simulink model "HWR"  (R2022b)
settings: Solver=ode23t  StartTime=0.0  StopTime=0.08  RelTol=1e-3
libraries: dspsigops x5, simulink x2, spsSeriesRLCBranchLib x2, spsVoltageMeasurementLib x2, spsACVoltageSourceLib x1, spsCurrentMeasurementLib x1, spspowerguiLib x1
settings Model: Creator=HP  LastModifiedBy=HP

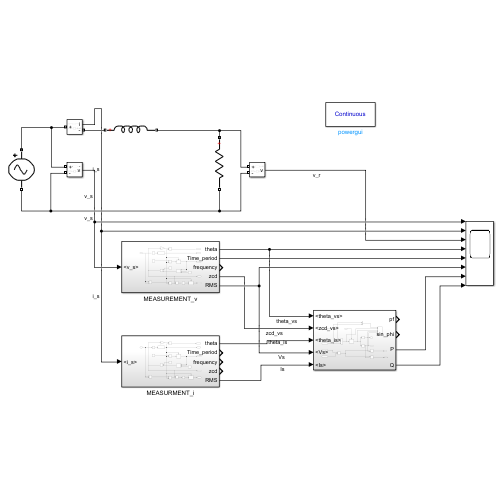
[thumbnail: Simulink's stored preview of the top-level diagram]
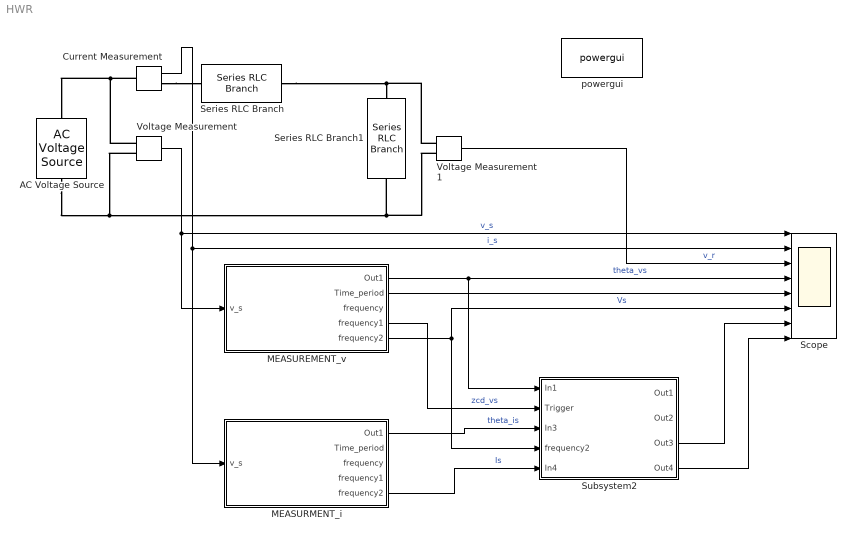
== system HWR ==
  AC Voltage Source : spsACVoltageSourceLib/AC Voltage Source  Amplitude=230*sqrt(2)  Phase=0  Frequency=1000  SampleTime=0  Measurements=None  BusType=swing  Pref=10e3  Qref=0  Qmin=-inf  Qmax=+inf
  Current Measurement : spsCurrentMeasurementLib/Current Measurement  PhasorSimulation=off  OutputType=Complex  PSBequivalent=0
  MEASUREMENT_v : Subsystem
  MEASURMENT_i : Subsystem
  Scope : Scope  NumInputPorts=8
  Series RLC Branch : spsSeriesRLCBranchLib/Series RLC Branch  LConnTagsString=__new0  RConnTagsString=__new0  BranchType=L  Resistance=1  Inductance=12.7e-3  SetiL0=off  InitialCurrent=0  Capacitance=1e-6  Setx0=off  InitialVoltage=0  Measurements=None
  Series RLC Branch1 : spsSeriesRLCBranchLib/Series RLC Branch  LConnTagsString=__new0  RConnTagsString=__new0  BranchType=R  Resistance=10  Inductance=12.7e-3  SetiL0=off  InitialCurrent=0  Capacitance=1e-6  Setx0=off  InitialVoltage=0  Measurements=None
  Subsystem2 : Subsystem
  Voltage Measurement : spsVoltageMeasurementLib/Voltage Measurement  PhasorSimulation=off  OutputType=Complex  PSBequivalent=0
  Voltage Measurement1 : spsVoltageMeasurementLib/Voltage Measurement  PhasorSimulation=off  OutputType=Complex  PSBequivalent=0
  powergui : spspowerguiLib/powergui  Priority=1  SimulationMode=Continuous  SampleTime=50e-6  frequency=60  Iterations=50  frequencyindice=1000  Pbase=100e6  ErrMax=1e-4  UnitsV=kV  UnitsW=MW  buscounter=0  FunctionMessages=off  echomessages=off  EnableUseOfTLC=off  CurrentSourceSwitches=off  DisableSnubberDevices=off  DisableRonSwitches=off  DisableVfSwitches=off  DisplayEquations=off  AutomaticDiscreteSolvers=off  SolverType=Tustin/Backward Euler (TBE)  Interpol=off  ExternalGateDelay=off  methode=off  Ts=100  x0status=blocks  SPID=on  SwTol=0  HookPort=off  NonlinearTolerance=1e-4  nMaxIteration=100  ContinueOnMaxIteration=off  RestoreLinks=warning  ResistiveCurrentMeasurement=off  Frange=[0:2:500]  Ylog=off  Xlog=on  ShowGrid=off  save=off  variable=ZData  structure=0  ZoomFFT=off  StartTime=0.0  cycles=1  DisplayStyle=1  fundamental=60  FreqAxis=off  MaxFrequency=1000  frequencyindicesteady=1  RmsSteady=1  display=off
  wires:
  Voltage Measurement/1 -> MEASUREMENT_v/1(v_s), Scope/1  "v_s"
  Current Measurement/1 -> MEASURMENT_i/1(v_s), Scope/2  "i_s"
  Voltage Measurement1/1 -> Scope/3  "v_r"
  MEASUREMENT_v/1(Out1) -> Subsystem2/1(In1), Scope/4  "theta_vs"
  MEASUREMENT_v/2(Time_period) -> Scope/5
  MEASUREMENT_v/5(frequency2) -> Subsystem2/4(frequency2), Scope/6  "Vs"
  MEASUREMENT_v/4(frequency1) -> Subsystem2/2(Trigger)  "zcd_vs"
  MEASURMENT_i/1(Out1) -> Subsystem2/3(In3)  "theta_is"
  MEASURMENT_i/5(frequency2) -> Subsystem2/5(In4)  "Is"
  Subsystem2/3(Out3) -> Scope/7
  Subsystem2/4(Out4) -> Scope/8
  connections:
  AC Voltage Source/LConn1 -- Voltage Measurement1/LConn2 -- Series RLC Branch1/RConn1 -- Voltage Measurement/LConn2
  Series RLC Branch/RConn1 -- Voltage Measurement1/LConn1 -- Series RLC Branch1/LConn1
  Current Measurement/RConn1 -- Series RLC Branch/LConn1
  Current Measurement/LConn1 -- Voltage Measurement/LConn1 -- AC Voltage Source/RConn1

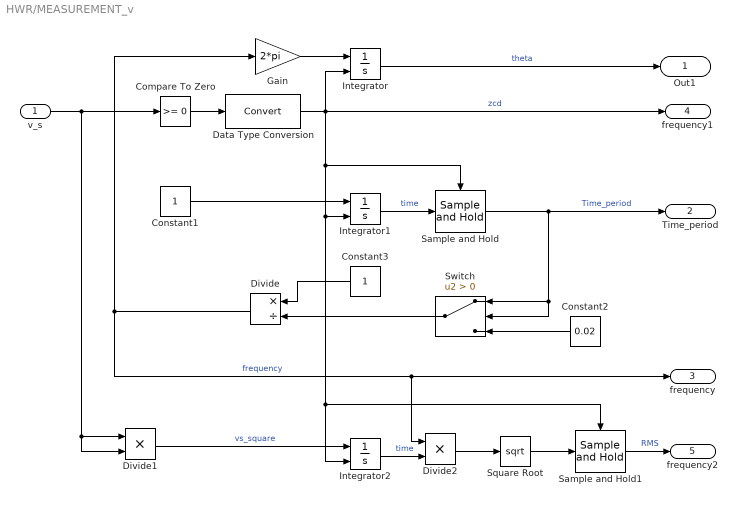
== system HWR/MEASUREMENT_v ==
  v_s : Inport
  Compare To Zero : simulink/Logic and Bit Operations/Compare To Zero  relop=>=  OutDataTypeStr=boolean
  Constant1 : Constant
  Constant2 : Constant  Value=0.02
  Constant3 : Constant
  Data Type Conversion : DataTypeConversion  SaturateOnIntegerOverflow=off  RndMeth=Floor
  Divide : Product  Inputs=*/
  Divide1 : Product  Inputs=**
  Divide2 : Product  Inputs=**
  Gain : Gain  Gain=2*pi
  Integrator : Integrator  ExternalReset=rising
  Integrator1 : Integrator  ExternalReset=rising
  Integrator2 : Integrator  ExternalReset=rising
  Sample and Hold : dspsigops/Sample and Hold  trig=Rising edge  initCond=0  latchinput=on
  Sample and Hold1 : dspsigops/Sample and Hold  trig=Rising edge  initCond=0  latchinput=on
  Square Root : Sqrt
  Switch : Switch  Criteria=u2 > Threshold  SaturateOnIntegerOverflow=off  InputSameDT=off
  Out1 : Outport
  Time_period : Outport  Port=2
  frequency : Outport  Port=3
  frequency1 : Outport  Port=4
  frequency2 : Outport  Port=5
  wires:
  Compare To Zero/1 -> Data Type Conversion/1
  Constant3/1 -> Divide/1
  Integrator/1 -> Out1/1  "theta"
  Divide/1 -> Gain/1, Divide2/1, frequency/1  "frequency"
  Data Type Conversion/1 -> Integrator1/2, Sample and Hold1/Trigger, Integrator2/2, Sample and Hold/Trigger, frequency1/1, Integrator/2  "zcd"
  Gain/1 -> Integrator/1
  Sample and Hold/1 -> Time_period/1, Switch/2, Switch/1  "Time_period"
  Constant2/1 -> Switch/3
  Constant1/1 -> Integrator1/1
  Integrator1/1 -> Sample and Hold/1  "time"
  Switch/1 -> Divide/2
  v_s/1 -> Divide1/2, Divide1/1, Compare To Zero/1
  Divide1/1 -> Integrator2/1  "vs_square"
  Integrator2/1 -> Divide2/2  "time"
  Divide2/1 -> Square Root/1
  Square Root/1 -> Sample and Hold1/1
  Sample and Hold1/1 -> frequency2/1  "RMS"

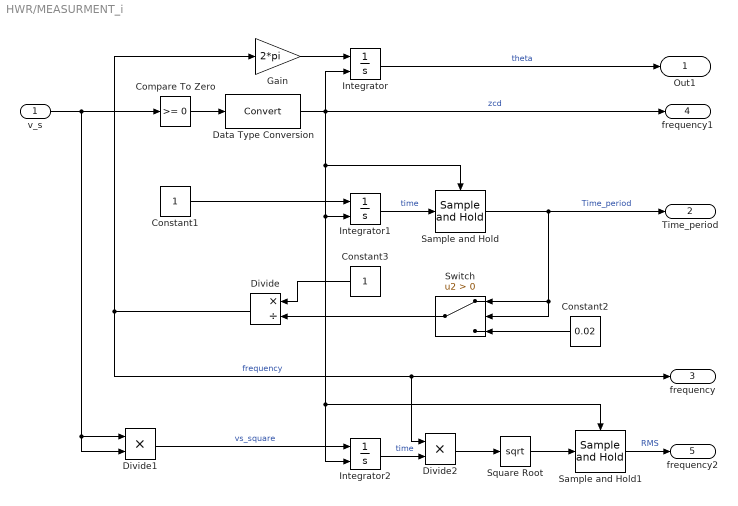
== system HWR/MEASURMENT_i ==
  v_s : Inport
  Compare To Zero : simulink/Logic and Bit Operations/Compare To Zero  relop=>=  OutDataTypeStr=boolean
  Constant1 : Constant
  Constant2 : Constant  Value=0.02
  Constant3 : Constant
  Data Type Conversion : DataTypeConversion  SaturateOnIntegerOverflow=off  RndMeth=Floor
  Divide : Product  Inputs=*/
  Divide1 : Product  Inputs=**
  Divide2 : Product  Inputs=**
  Gain : Gain  Gain=2*pi
  Integrator : Integrator  ExternalReset=rising
  Integrator1 : Integrator  ExternalReset=rising
  Integrator2 : Integrator  ExternalReset=rising
  Sample and Hold : dspsigops/Sample and Hold  trig=Rising edge  initCond=0  latchinput=on
  Sample and Hold1 : dspsigops/Sample and Hold  trig=Rising edge  initCond=0  latchinput=on
  Square Root : Sqrt
  Switch : Switch  Criteria=u2 > Threshold  SaturateOnIntegerOverflow=off  InputSameDT=off
  Out1 : Outport
  Time_period : Outport  Port=2
  frequency : Outport  Port=3
  frequency1 : Outport  Port=4
  frequency2 : Outport  Port=5
  wires:
  Sample and Hold1/1 -> frequency2/1  "RMS"
  Square Root/1 -> Sample and Hold1/1
  Divide2/1 -> Square Root/1
  Integrator2/1 -> Divide2/2  "time"
  Divide1/1 -> Integrator2/1  "vs_square"
  v_s/1 -> Compare To Zero/1, Divide1/1, Divide1/2
  Switch/1 -> Divide/2
  Integrator1/1 -> Sample and Hold/1  "time"
  Constant1/1 -> Integrator1/1
  Constant2/1 -> Switch/3
  Sample and Hold/1 -> Switch/1, Switch/2, Time_period/1  "Time_period"
  Gain/1 -> Integrator/1
  Data Type Conversion/1 -> Integrator/2, frequency1/1, Sample and Hold/Trigger, Integrator2/2, Sample and Hold1/Trigger, Integrator1/2  "zcd"
  Divide/1 -> frequency/1, Divide2/1, Gain/1  "frequency"
  Integrator/1 -> Out1/1  "theta"
  Constant3/1 -> Divide/1
  Compare To Zero/1 -> Data Type Conversion/1

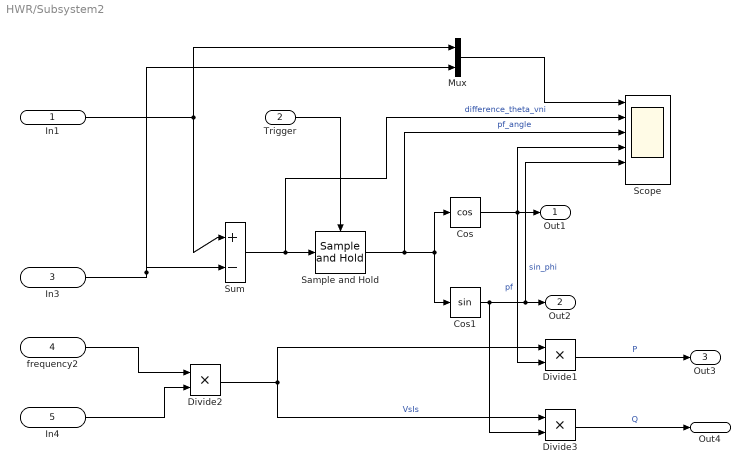
== system HWR/Subsystem2 ==
  In1 : Inport
  Trigger : Inport  Port=2
  In3 : Inport  Port=3
  frequency2 : Inport  Port=4
  In4 : Inport  Port=5
  Cos : Trigonometry  Operator=cos
  Cos1 : Trigonometry
  Divide1 : Product  Inputs=**
  Divide2 : Product  Inputs=**
  Divide3 : Product  Inputs=**
  Mux : Mux  Inputs=2
  Sample and Hold : dspsigops/Sample and Hold  trig=Rising edge  initCond=0  latchinput=on
  Scope : Scope  NumInputPorts=6
  Sum : Sum  Inputs=|+-
  Out1 : Outport
  Out2 : Outport  Port=2
  Out3 : Outport  Port=3
  Out4 : Outport  Port=4
  wires:
  In3/1 -> Mux/2, Sum/2
  Cos/1 -> Divide1/2, Scope/4, Out1/1  "pf"
  Sample and Hold/1 -> Scope/3, Cos1/1, Cos/1  "pf_angle"
  Trigger/1 -> Sample and Hold/Trigger
  Cos1/1 -> Divide3/2, Scope/5, Out2/1  "sin_phi"
  Sum/1 -> Scope/2, Sample and Hold/1  "difference_theta_vni"
  In1/1 -> Sum/1, Mux/1
  Mux/1 -> Scope/1
  frequency2/1 -> Divide2/1
  In4/1 -> Divide2/2
  Divide2/1 -> Divide3/1, Divide1/1  "VsIs"
  Divide1/1 -> Out3/1  "P"
  Divide3/1 -> Out4/1  "Q"
